simulink model "model_observer_noise"  (R2024a)
settings: Solver=FixedStepAuto  StartTime=0.0  StopTime=10.0  FixedStep=0.0001  RelTol=1e-3
undefined symbols (not defined in the file): A, C, L, white_noise_var, x0, x_hat0
libraries: dspsrcs4 x1
settings Model: Creator=anton  LastModifiedBy=anton

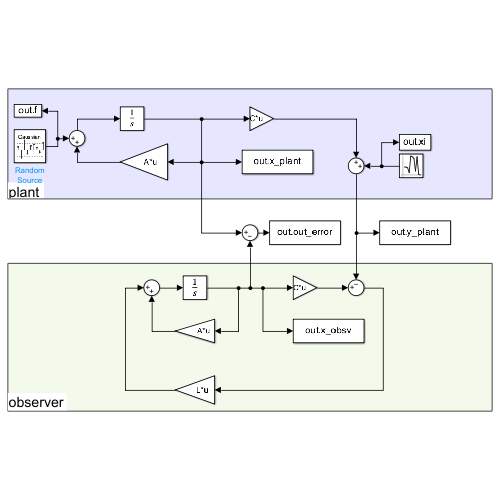
[thumbnail: Simulink's stored preview of the top-level diagram]
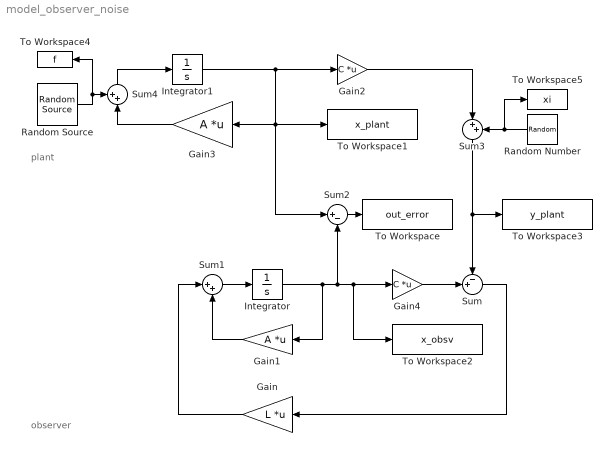
== system model_observer_noise ==
  note: observer
  note: plant
  Gain : Gain  Gain=L  Multiplication=Matrix(K*u)
  Gain1 : Gain  Gain=A  Multiplication=Matrix(K*u)
  Gain2 : Gain  Gain=C  Multiplication=Matrix(K*u)
  Gain3 : Gain  Gain=A  Multiplication=Matrix(K*u)
  Gain4 : Gain  Gain=C  Multiplication=Matrix(K*u)
  Integrator : Integrator  InitialCondition=x_hat0
  Integrator1 : Integrator  InitialCondition=x0
  Random Number : RandomNumber  Variance=white_noise_var  SampleTime=0.0001
  Random Source : dspsrcs4/Random Source  SrcType=Gaussian  MinVal=uniform_min  MaxVal=uniform_max  MeanVal=0  VarVal=4  RepMode=Specify seed  rawSeed=1  IsInherit=off  SampTime=0.0001  SampFrame=1  OutComplex=Real  DataType=double  SimulateUsing=Interpreted execution
  Sum : Sum  Inputs=-+|
  Sum1 : Sum  Inputs=|++
  Sum2 : Sum  Inputs=|+-
  Sum3 : Sum  Inputs=|++
  Sum4 : Sum  Inputs=++|
  To Workspace : ToWorkspace  VariableName=out_error  SaveFormat=Timeseries  SampleTime=-1
  To Workspace1 : ToWorkspace  VariableName=x_plant  SaveFormat=Timeseries  SampleTime=-1
  To Workspace2 : ToWorkspace  VariableName=x_obsv  SaveFormat=Timeseries  SampleTime=-1
  To Workspace3 : ToWorkspace  VariableName=y_plant  SaveFormat=Timeseries  SampleTime=-1
  To Workspace4 : ToWorkspace  VariableName=f  SaveFormat=Timeseries  SampleTime=-1
  To Workspace5 : ToWorkspace  VariableName=xi  SaveFormat=Timeseries  SampleTime=-1
  wires:
  Sum/1 -> Gain/1
  Gain/1 -> Sum1/1
  Gain1/1 -> Sum1/2
  Sum1/1 -> Integrator/1
  Integrator/1 -> Gain1/1, Sum2/2, To Workspace2/1, Gain4/1
  Integrator1/1 -> Sum2/1, To Workspace1/1, Gain3/1, Gain2/1
  Gain4/1 -> Sum/2
  Sum2/1 -> To Workspace/1
  Gain2/1 -> Sum3/1
  Sum3/1 -> To Workspace3/1, Sum/1
  Random Number/1 -> To Workspace5/1, Sum3/2
  Gain3/1 -> Sum4/2
  Sum4/1 -> Integrator1/1
  Random Source/1 -> To Workspace4/1, Sum4/1
